simulink model "transport_tester"  (R2024b)
settings: Solver=VariableStepAuto  StartTime=0.0  StopTime=10.0  RelTol=1e-3
libraries: transport_lib x1
settings Model: Creator=marcv  LastModifiedBy=marcv

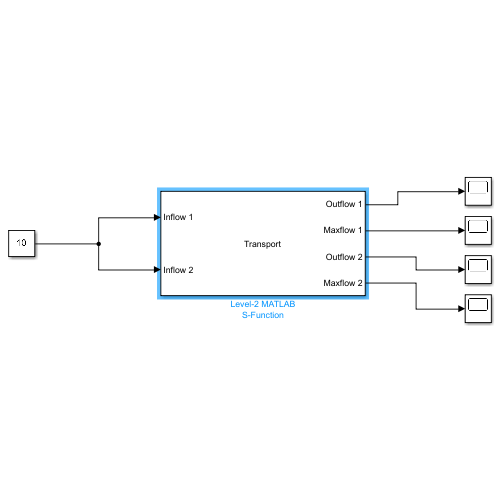
[thumbnail: Simulink's stored preview of the top-level diagram]
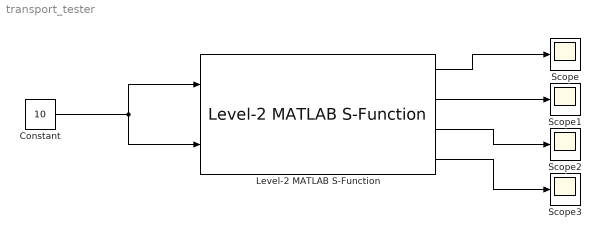
== system transport_tester ==
  Constant : Constant  Value=10
  Level-2 MATLAB S-Function : transport_lib/Level-2 MATLAB S-Function  max_flow_result1=88.401  max_flow_result2=0  flowDirec=Bidirectional  setupopt=Transport only  Transporttype=Pipeline  Dist=20000  elevation=2  width=1  depth=3  diameter=0.2  dP=5  customflow=0  filteroption=Common filter  Fflowmax=3000  dPfilter=1  selectedfilter=Sand [90 m3/h (UDI 4U4604)]  filterparallel=1
  Scope{,1..3} (4 alike) : Scope
  wires:
  Constant/1 -> Level-2 MATLAB S-Function/2, Level-2 MATLAB S-Function/1
  Level-2 MATLAB S-Function/1 -> Scope/1
  Level-2 MATLAB S-Function/2 -> Scope1/1
  Level-2 MATLAB S-Function/3 -> Scope2/1
  Level-2 MATLAB S-Function/4 -> Scope3/1
